simulink model "ME419_Ex1_2"  (R2023b)
settings: Solver=VariableStepAuto  StartTime=0.0  StopTime=10.0  RelTol=1e-6
settings Model: Creator=aliawolken  LastModifiedBy=aliawolken

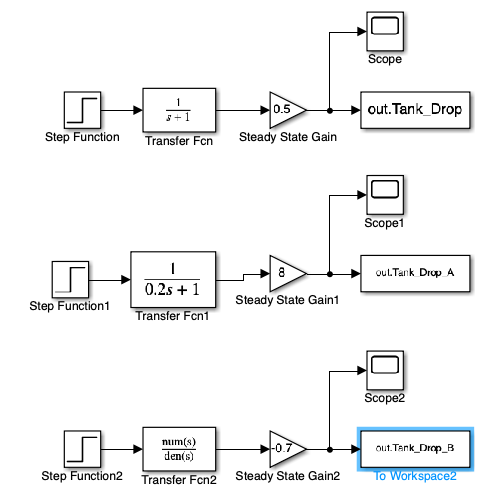
[thumbnail: Simulink's stored preview of the top-level diagram]
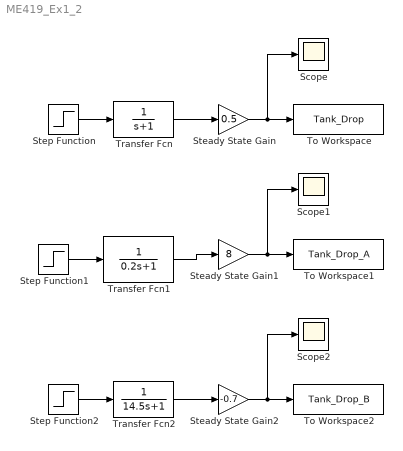
== system ME419_Ex1_2 ==
  Scope : Scope
  Scope1 : Scope
  Scope2 : Scope
  Steady State Gain : Gain  Gain=0.5
  Steady State Gain1 : Gain  Gain=8
  Steady State Gain2 : Gain  Gain=-0.7
  Step Function : Step  SampleTime=0
  Step Function1 : Step  SampleTime=0
  Step Function2 : Step  SampleTime=0
  To Workspace : ToWorkspace  VariableName=Tank_Drop  SampleTime=-1
  To Workspace1 : ToWorkspace  VariableName=Tank_Drop_A  SampleTime=-1
  To Workspace2 : ToWorkspace  VariableName=Tank_Drop_B  SampleTime=-1
  Transfer Fcn : TransferFcn  Denominator=[1 1]
  Transfer Fcn1 : TransferFcn  Denominator=[0.2 1]
  Transfer Fcn2 : TransferFcn  Denominator=[14.5 1]
  wires:
  Step Function/1 -> Transfer Fcn/1
  Transfer Fcn/1 -> Steady State Gain/1
  Steady State Gain/1 -> Scope/1, To Workspace/1
  Steady State Gain1/1 -> Scope1/1, To Workspace1/1
  Transfer Fcn1/1 -> Steady State Gain1/1
  Step Function1/1 -> Transfer Fcn1/1
  Step Function2/1 -> Transfer Fcn2/1
  Transfer Fcn2/1 -> Steady State Gain2/1
  Steady State Gain2/1 -> Scope2/1, To Workspace2/1
